simulink model "xiti4_2"  (Simulink 5.0)
settings: Solver=ode45  SolverMode=SingleTasking  StartTime=0.0  StopTime=2  FixedStep=0.2  RelTol=1e-3
settings Model: LastModifiedBy=ThinkPad

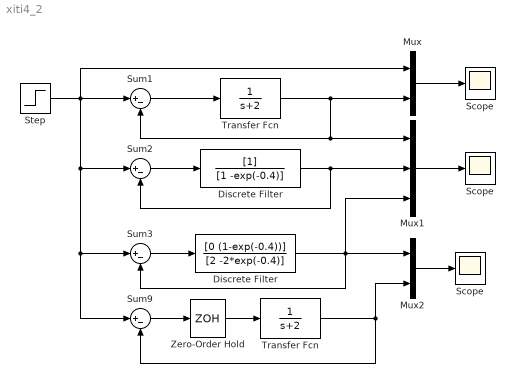
== system xiti4_2 ==
  " Scope " : Scope
      settings: YMin=-3.5  YMax=1  SaveName=ScopeData3  MaxDataPoints=500000
  Discrete Filter : DiscreteFilter  Denominator=[1 -exp(-0.4)]  SampleTime=0.2
  "Discrete Filter " : DiscreteFilter  Numerator=[0 (1-exp(-0.4))]  Denominator=[2 -2*exp(-0.4)]  SampleTime=0.2
  Mux : Mux  Inputs=2
  Mux1 : Mux  Inputs=3
  Mux2 : Mux  Inputs=2
  Scope : Scope
      settings: YMin=-3.5  YMax=1  SaveName=ScopeData2  MaxDataPoints=500000
  "Scope " : Scope
      settings: YMin=-3.5  YMax=1  MaxDataPoints=500000
  "Step " : Step  Time=0  SampleTime=0
  Sum{1..3,9} (4 alike) : Sum  Inputs=|+-  SaturateOnIntegerOverflow=on
  "Transfer Fcn " : TransferFcn  Denominator=[1 2]
  "Transfer Fcn  " : TransferFcn  Denominator=[1 2]
  "Zero-Order Hold  " : ZeroOrderHold  SampleTime=0.2
  wires:
  Sum1/1 -> "Transfer Fcn "/1
  Mux/1 -> "Scope "/1
  "Transfer Fcn "/1 -> Mux/2, Sum1/2, Mux1/1
  Sum2/1 -> Discrete Filter/1
  Mux1/1 -> Scope/1
  Sum3/1 -> "Discrete Filter "/1
  Mux2/1 -> " Scope "/1
  "Discrete Filter "/1 -> Sum3/2, Mux1/3, Mux2/1
  "Transfer Fcn  "/1 -> Sum9/2, Mux2/2
  "Zero-Order Hold  "/1 -> "Transfer Fcn  "/1
  Sum9/1 -> "Zero-Order Hold  "/1
  "Step "/1 -> Sum1/1, Sum2/1, Sum3/1, Sum9/1, Mux/1
  Discrete Filter/1 -> Mux1/2, Sum2/2
